simulink model "BlockDiagram"  (R2025b)
settings: Solver=VariableStepAuto  StartTime=0.0  StopTime=10.0  RelTol=1e-3
values from neighbouring files (symbols this model uses):
  P_amb = 101325    [init_engine_params.m]
  rho_f = 789    [init_engine_params.m]
  rho_ox = 988.82    [init_engine_params.m]
  V_c = 2.5335373958699e-4    (= 0.000253353739587)    [init_engine_params.m]
undefined symbols (not defined in the file or in its folder): CdA_max_f, CdA_max_ox, P_feed_f, P_feed_ox
settings Model: Creator=gruby  LastModifiedBy=gruby

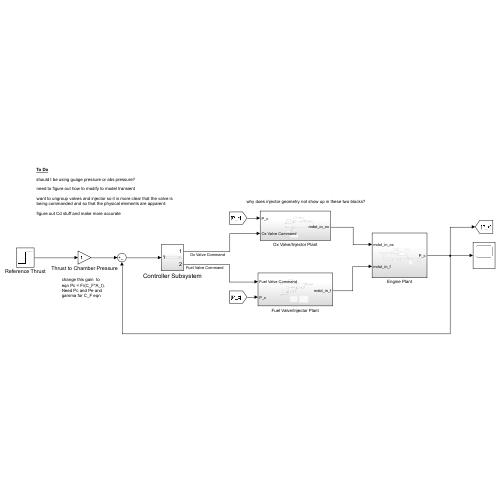
[thumbnail: Simulink's stored preview of the top-level diagram]
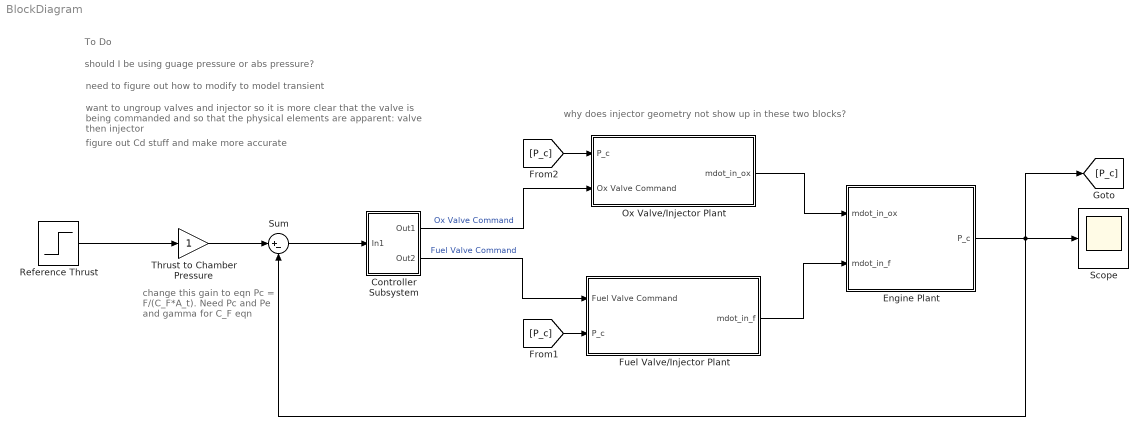
== system BlockDiagram ==
  note: figure out Cd stuff and make more accurate
  note: To Do
  note: need to figure out how to modify to model transient
  note: want to ungroup valves and injector so it is more clear that the valve is being commanded and so that the physical elements are apparent: valve then injector
  note: why does injector geometry not show up in these two blocks?
  note: should I be using guage pressure or abs pressure?
  note: change this gain to eqn Pc = F/(C_F*A_t). Need Pc and Pe and gamma for C_F eqn
  Controller Subsystem : Subsystem
  Engine Plant : Subsystem
  Fuel Valve/Injector Plant : Subsystem
  Ox Valve/Injector Plant : Subsystem
  Reference Thrust : Step  SampleTime=0
  Scope : Scope
      settings: ActiveDisplayYMinimum=-1.8374784378622904  ActiveDisplayYMaximum=16.537497604206919
  Sum : Sum  Inputs=|+-
  Thrust to Chamber Pressure : Gain
  wires:
  Sum/1 -> Controller Subsystem/1(In1)
  Thrust to Chamber Pressure/1 -> Sum/1
  Reference Thrust/1 -> Thrust to Chamber Pressure/1
  Engine Plant/1(P_c) -> Scope/1, [P_c], Sum/2
  [P_c] -> Ox Valve/Injector Plant/1(P_c)
  Controller Subsystem/1(Out1) -> Ox Valve/Injector Plant/2(Ox Valve Command)  "Ox Valve Command"
  Ox Valve/Injector Plant/1(mdot_in_ox) -> Engine Plant/1(mdot_in_ox)
  Controller Subsystem/2(Out2) -> Fuel Valve/Injector Plant/1(Fuel Valve Command)  "Fuel Valve Command"
  [P_c] -> Fuel Valve/Injector Plant/2(P_c)
  Fuel Valve/Injector Plant/1(mdot_in_f) -> Engine Plant/2(mdot_in_f)

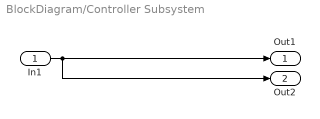
== system BlockDiagram/Controller Subsystem ==
  In1 : Inport
  Out1 : Outport
  Out2 : Outport  Port=2
  wires:
  In1/1 -> Out2/1, Out1/1

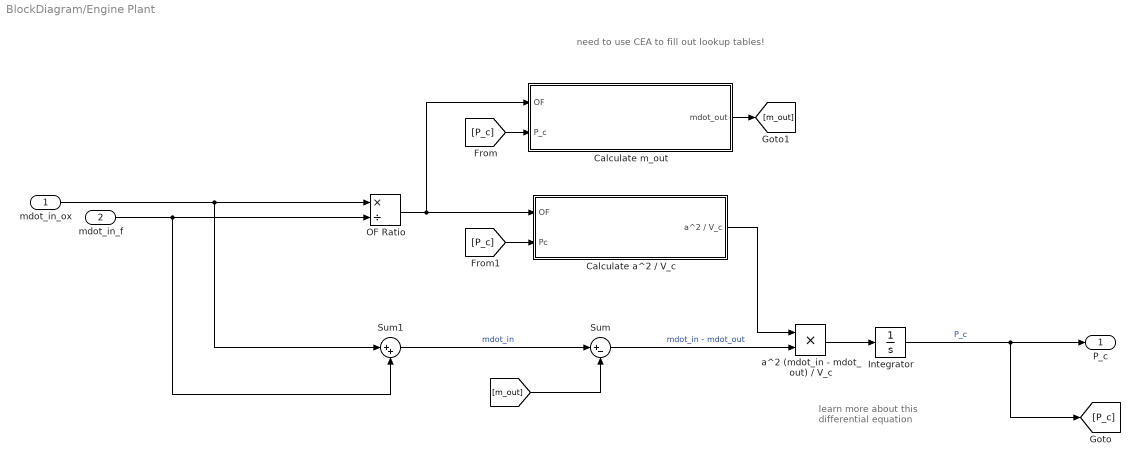
== system BlockDiagram/Engine Plant ==
  note: need to use CEA to fill out lookup tables!
  note: learn more about this differential equation
  mdot_in_ox : Inport
  mdot_in_f : Inport  Port=2
  Calculate a^2 / V_c : Subsystem
  Calculate m_out : Subsystem
  Integrator : Integrator  InitialCondition=P_amb
  OF Ratio : Product  Inputs=*/
  Sum : Sum  Inputs=|+-
  Sum1 : Sum  Inputs=|++
  "a^2 (mdot_in - mdot_out) / V_c " : Product
  P_c : Outport
  wires:
  mdot_in_f/1 -> Sum1/2, OF Ratio/2
  mdot_in_ox/1 -> Sum1/1, OF Ratio/1
  Sum/1 -> "a^2 (mdot_in - mdot_out) / V_c "/2  "mdot_in - mdot_out"
  Integrator/1 -> P_c/1, [P_c]  "P_c"
  OF Ratio/1 -> Calculate m_out/1(OF), Calculate a^2 / V_c/1(OF)
  Sum1/1 -> Sum/1  "mdot_in"
  "a^2 (mdot_in - mdot_out) / V_c "/1 -> Integrator/1
  [P_c] -> Calculate m_out/2(P_c)
  [P_c] -> Calculate a^2 / V_c/2(Pc)
  Calculate a^2 / V_c/1(a^2 / V_c) -> "a^2 (mdot_in - mdot_out) / V_c "/1
  Calculate m_out/1(mdot_out) -> [m_out]
  [m_out] -> Sum/2

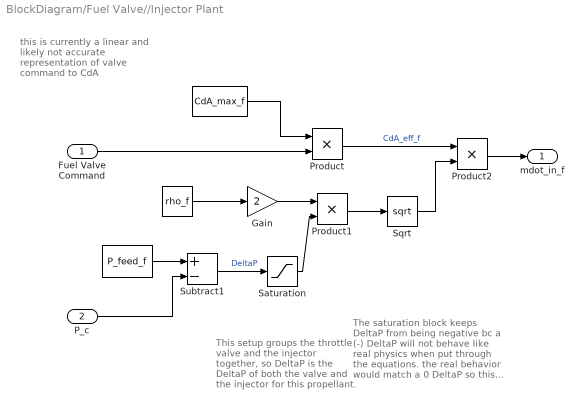
== system BlockDiagram/Fuel Valve//Injector Plant ==
  note: This setup groups the throttle valve and the injector together, so DeltaP is the DeltaP of both the valve and the injector for this propellant.
  note: The saturation block keeps DeltaP from being negative bc a (-) DeltaP will not behave like real physics when put through the equations. the real behavior would match a 0 DeltaP so this makes a lower lim of 0.
  note: this is currently a linear and likely not accurate representation of valve command to CdA
  Fuel Valve Command : Inport
  P_c : Inport  Port=2
  " " : Constant  Value=P_feed_f
  "  " : Constant  Value=rho_f
  "   " : Constant  Value=CdA_max_f
  Gain : Gain  Gain=2
  Product : Product
  Product1 : Product
  Product2 : Product
  Saturation : Saturate  LowerLimit=0
  Sqrt : Sqrt
  Subtract1 : Sum  Inputs=+-
  mdot_in_f : Outport
  wires:
  Gain/1 -> Product1/1
  Product/1 -> Product2/1  "CdA_eff_f"
  Subtract1/1 -> Saturation/1  "DeltaP"
  " "/1 -> Subtract1/1
  "  "/1 -> Gain/1
  Saturation/1 -> Product1/2
  Product1/1 -> Sqrt/1
  Sqrt/1 -> Product2/2
  P_c/1 -> Subtract1/2
  Product2/1 -> mdot_in_f/1
  Fuel Valve Command/1 -> Product/2
  "   "/1 -> Product/1

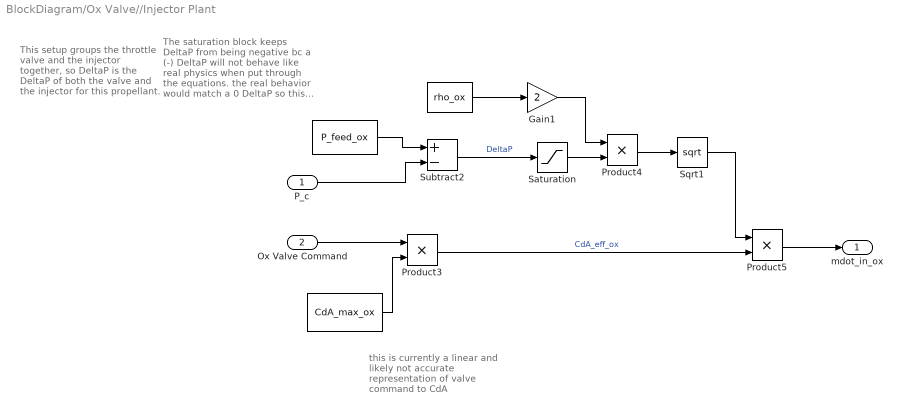
== system BlockDiagram/Ox Valve//Injector Plant ==
  note: This setup groups the throttle valve and the injector together, so DeltaP is the DeltaP of both the valve and the injector for this propellant.
  note: The saturation block keeps DeltaP from being negative bc a (-) DeltaP will not behave like real physics when put through the equations. the real behavior would match a 0 DeltaP so this makes a lower lim of 0.
  note: this is currently a linear and likely not accurate representation of valve command to CdA
  P_c : Inport
  Ox Valve Command : Inport  Port=2
  " " : Constant  Value=CdA_max_ox
  "  " : Constant  Value=P_feed_ox
  "   " : Constant  Value=rho_ox
  Gain1 : Gain  Gain=2
  Product3 : Product
  Product4 : Product
  Product5 : Product
  Saturation : Saturate  LowerLimit=0
  Sqrt1 : Sqrt
  Subtract2 : Sum  Inputs=+-
  mdot_in_ox : Outport
  wires:
  Saturation/1 -> Product4/2
  "   "/1 -> Gain1/1
  Subtract2/1 -> Saturation/1  "DeltaP"
  "  "/1 -> Subtract2/1
  Gain1/1 -> Product4/1
  Product5/1 -> mdot_in_ox/1
  " "/1 -> Product3/2
  Product4/1 -> Sqrt1/1
  Ox Valve Command/1 -> Product3/1
  P_c/1 -> Subtract2/2
  Sqrt1/1 -> Product5/1
  Product3/1 -> Product5/2  "CdA_eff_ox"

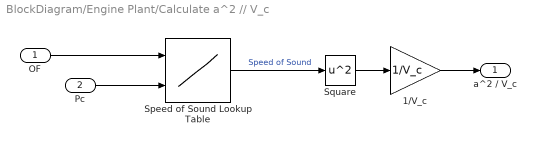
== system BlockDiagram/Engine Plant/Calculate a^2 // V_c ==
  OF : Inport
  Pc : Inport  Port=2
  1/V_c : Gain  Gain=1/V_c
  Speed of Sound Lookup Table : Lookup_n-D  BreakpointsForDimension1=[1:3]  BreakpointsForDimension2=[1:3]  InternalRulePriority=Speed  RndMeth=Simplest
      settings: InputPortMap=u0,u1
  Square : Math  Operator=square
  a^2 / V_c : Outport
  wires:
  Speed of Sound Lookup Table/1 -> Square/1  "Speed of Sound"
  OF/1 -> Speed of Sound Lookup Table/1
  Square/1 -> 1/V_c/1
  Pc/1 -> Speed of Sound Lookup Table/2
  1/V_c/1 -> a^2 / V_c/1

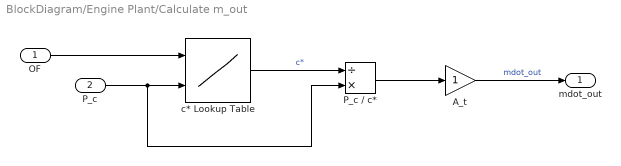
== system BlockDiagram/Engine Plant/Calculate m_out ==
  OF : Inport
  P_c : Inport  Port=2
  A_t : Gain
  P_c / c* : Product  Inputs=/*
  c* Lookup Table : Lookup_n-D  BreakpointsForDimension1=[1:3]  BreakpointsForDimension2=[1:3]  InternalRulePriority=Speed  RndMeth=Simplest
      settings: InputPortMap=u0,u1
  mdot_out : Outport
  wires:
  c* Lookup Table/1 -> P_c / c*/1  "c*"
  P_c / c*/1 -> A_t/1
  OF/1 -> c* Lookup Table/1
  A_t/1 -> mdot_out/1  "mdot_out"
  P_c/1 -> P_c / c*/2, c* Lookup Table/2
